simulink model "suavizado_step"  (R2018b)
settings: Solver=VariableStepAuto  StartTime=0.0  StopTime=1000  RelTol=1e-3
undefined symbols (not defined in the file or in its folder): tau_smooth
libraries: simulink_extras x4
settings Model: Creator=simon  LastModifiedBy=simon

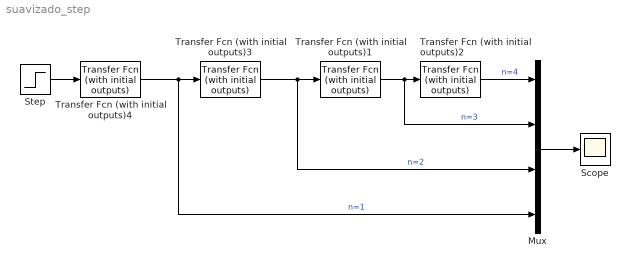
== system suavizado_step ==
  Mux : Mux
  Scope : Scope
  Step : Step  Time=50  SampleTime=0
  Transfer Fcn (with initial outputs){1..4} (4 alike) : simulink_extras/Additional Linear/Transfer Fcn (with initial outputs)  N=[1]  D="[tau_smooth  1]"  Y0=0  U0=0
  wires:
  Step/1 -> Transfer Fcn (with initial outputs)4/1
  Transfer Fcn (with initial outputs)4/1 -> Mux/4, Transfer Fcn (with initial outputs)3/1  "n=1"
  Transfer Fcn (with initial outputs)2/1 -> Mux/1  "n=4"
  Transfer Fcn (with initial outputs)1/1 -> Mux/2, Transfer Fcn (with initial outputs)2/1  "n=3"
  Transfer Fcn (with initial outputs)3/1 -> Mux/3, Transfer Fcn (with initial outputs)1/1  "n=2"
  Mux/1 -> Scope/1
